simulink model "DC_Charging_Sequence_Block"  (R2025b)
settings: Solver=VariableStepAuto  StartTime=0.0  StopTime=10.0  RelTol=1e-3
settings Model: Creator=noahm  LastModifiedBy=noahm

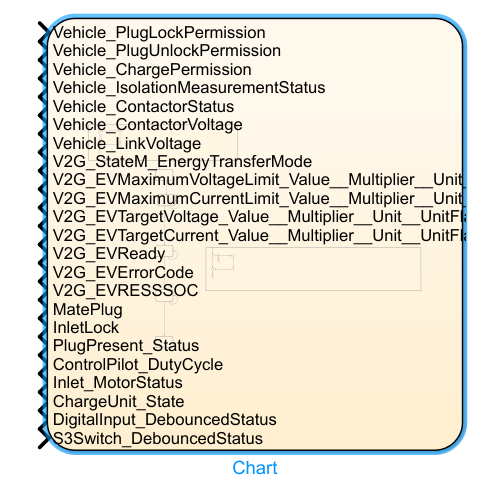
[thumbnail: Simulink's stored preview of the top-level diagram]
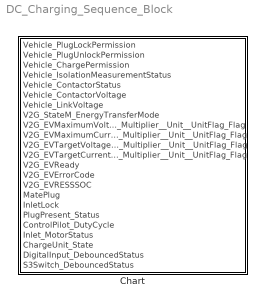
== system DC_Charging_Sequence_Block ==
  Chart : Stateflow chart  TreatAsAtomicUnit=on

== stateflow chart DC_Charging_Sequence_Block/Chart ==
  state PlugMated=MateLogic(in1, in2, in3, in4) [function]
    (junction 67) -> (junction 68) [order 1] : [Vehicle_PlugLockPermissio == 1 && PlugPresent_Status >= 2 && ControlPilot_DutyCycle >= 2 && Inlet_MotorStatus == 0]
    (junction 68) -> (junction 70) : {PlugMated == 1;}
    (junction 67) -> (junction 69) [order 2] : {PlugMated == 0;}
    (default) -> (junction 55)
    (junction 70) -> (junction 69)
    (junction 69) -> (junction 71)
  state DC01
    nletsLock=0;
  state DC02
    nletsLock=0;
  state DC03
  state DC4Check=DC4Logic(in1, in2, in3, in4, in5) [function]
    (default) -> (junction 84)
    (junction 101) -> (junction 102) [order 1] : [ControlPilot_DutyCycle <= 7 && ControlPilot_DutyCycle >=3 && Inlet_MotorStatus == 1 && ChargeUnit_State == 314 && DigitalInput_DebouncedStatus == 0 && S3Switch_DebouncedStatus == 0]
    (junction 101) -> (junction 103) [order 2] : {DC4Check == 0;}
    (junction 102) -> (junction 104) : {DC4Check == 1;}
    (junction 104) -> (junction 103)
    (junction 103) -> (junction 105)
  state DC04
  state DC05
  (default) -> (junction 67) [order 2]
  (default) -> DC01 [order 1]
  DC01 -> DC02 : [MatePlug==1]
  DC02 -> DC02 [order 2] : [~MateLogic(Vehicle_PlugLockPermission, PlugPresent_Status, ControlPilot_DutyCycle, Inlet_MotorStatus)]
  DC02 -> DC03 [order 1] : [MateLogic(Vehicle_PlugLockPermission, PlugPresent_Status, ControlPilot_DutyCycle, Inlet_MotorStatus)]
  (default) -> (junction 101) [order 3]
  DC03 -> DC03 [order 2] : [~InletLock]
  DC03 -> DC04 [order 1] : [InletLock]
  DC04 -> DC04 [order 2] : [~DC4Check(ControlPilot_DutyCycle, CycleInlet_MotorStatus, ChargeUnit_State, DigitalInput_DebouncedStatus, S3Switch_DebouncedStatus)]
  DC04 -> DC05 [order 1] : [DC4Check(ControlPilot_DutyCycle, CycleInlet_MotorStatus, ChargeUnit_State, DigitalInput_DebouncedStatus, S3Switch_DebouncedStatus)]
  data: PlugMated function_output; in1 function_input; in2 function_input; in3 function_input; in4 function_input; DC4Check function_output; in1 function_input; in2 function_input; in3 function_input; in4 function_input; in5 function_input; Vehicle_PlugLockPermission input; Vehicle_PlugUnlockPermission input; Vehicle_ChargePermission input; Vehicle_IsolationMeasurementStatus input; Vehicle_ContactorStatus input; Vehicle_ContactorVoltage input; Vehicle_LinkVoltage input; V2G_StateM_EnergyTransferMode input; V2G_EVMaximumVoltageLimit_Value__Multiplier__Unit__UnitFlag_Flag input; V2G_EVMaximumCurrentLimit_Value__Multiplier__Unit__UnitFlag_Flag input; V2G_EVTargetVoltage_Value__Multiplier__Unit__UnitFlag_Flag input; V2G_EVTargetCurrent_Value__Multiplier__Unit__UnitFlag_Flag input; V2G_EVReady input; V2G_EVErrorCode input; V2G_EVRESSSOC input; MatePlug input; InletLock input; PlugPresent_Status input; ControlPilot_DutyCycle input; Inlet_MotorStatus input; ChargeUnit_State input; DigitalInput_DebouncedStatus input; S3Switch_DebouncedStatus input
